simulink subsystem "GenericModulation"  (R2024a)
settings: Solver=VariableStepAuto  StartTime=0.0  StopTime=10.0  RelTol=1e-3
settings Model: Creator=dfurodet  LastModifiedBy=dfurodet

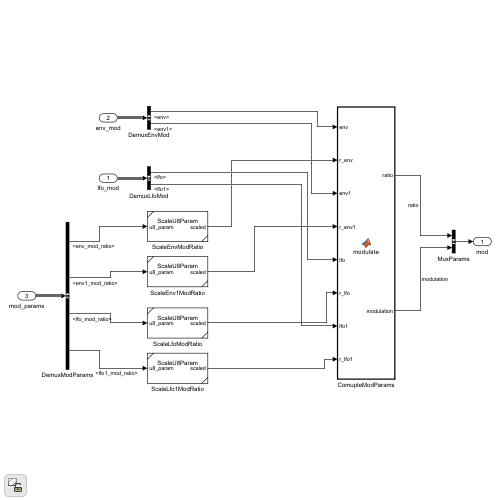
[thumbnail: Simulink's stored preview of the top-level diagram]
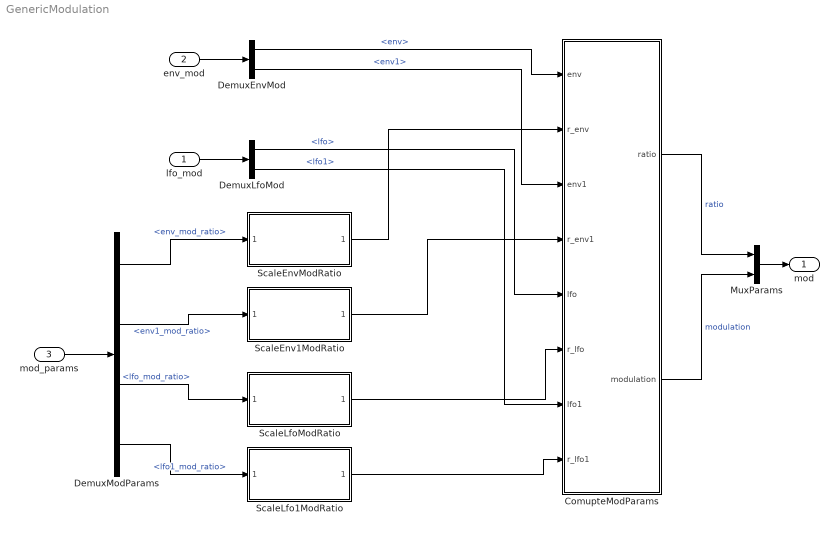
== system GenericModulation ==
  lfo_mod : Inport
  env_mod : Inport  Port=2
  mod_params : Inport  Port=3
  ComupteModParams : MATLAB Function  TreatAsAtomicUnit=on
  DemuxEnvMod : BusSelector  OutputSignals=env,env1
  DemuxLfoMod : BusSelector  OutputSignals=lfo,lfo1
  DemuxModParams : BusSelector  OutputSignals=env_mod_ratio,env1_mod_ratio,lfo_mod_ratio,lfo1_mod_ratio
  MuxParams : BusCreator  Inputs=2
  ScaleEnv1ModRatio : Subsystem  ReferencedSubsystem=ScaleU8Param
  ScaleEnvModRatio : Subsystem  ReferencedSubsystem=ScaleU8Param
  ScaleLfo1ModRatio : Subsystem  ReferencedSubsystem=ScaleU8Param
  ScaleLfoModRatio : Subsystem  ReferencedSubsystem=ScaleU8Param
  mod : Outport
  wires:
  mod_params/1 -> DemuxModParams/1
  DemuxModParams/1 -> ScaleEnvModRatio/1  "<env_mod_ratio>"
  DemuxModParams/2 -> ScaleEnv1ModRatio/1  "<env1_mod_ratio>"
  DemuxModParams/3 -> ScaleLfoModRatio/1  "<lfo_mod_ratio>"
  DemuxModParams/4 -> ScaleLfo1ModRatio/1  "<lfo1_mod_ratio>"
  env_mod/1 -> DemuxEnvMod/1
  lfo_mod/1 -> DemuxLfoMod/1
  DemuxEnvMod/1 -> ComupteModParams/1(env)  "<env>"
  DemuxEnvMod/2 -> ComupteModParams/3(env1)  "<env1>"
  DemuxLfoMod/1 -> ComupteModParams/5(lfo)  "<lfo>"
  DemuxLfoMod/2 -> ComupteModParams/7(lfo1)  "<lfo1>"
  ScaleEnvModRatio/1 -> ComupteModParams/2(r_env)
  ScaleEnv1ModRatio/1 -> ComupteModParams/4(r_env1)
  ScaleLfoModRatio/1 -> ComupteModParams/6(r_lfo)
  ScaleLfo1ModRatio/1 -> ComupteModParams/8(r_lfo1)
  ComupteModParams/1(ratio) -> MuxParams/1  "ratio"
  ComupteModParams/2(modulation) -> MuxParams/2  "modulation"
  MuxParams/1 -> mod/1

== matlab function GenericModulation/ComupteModParams ==
  data: env input; ratio output; r_env input; env1 input; r_env1 input; lfo input; r_lfo input; lfo1 input; r_lfo1 input; modulation output
function [ratio, modulation] = modulate(env, r_env, env1, r_env1, lfo, r_lfo, lfo1, r_lfo1)
% s is the total amount of modulation
ratio = r_env + r_env1 + r_lfo + r_lfo1;
if ratio == 0
    modulation = single(0);
else
    % Rescale every modulation source according to its actual weight
    a_env = env * r_env / ratio;
    a_env1 = env1 * r_env1 / ratio;
    a_lfo = lfo * r_lfo / ratio;
    a_lfo1 = lfo1 * r_lfo1 / ratio;
    % Remove the amount of modulation from the initial signal and modulate
    % this amount with modulation sources
    % The modulation result for a signal S is S*(1 - s + m)
    modulation = a_env * env + a_env1 * env1 + a_lfo * lfo + a_lfo1 * lfo1;
end
